simulink model "Project1_week3_sim"  (R2023b)
settings: Solver=VariableStepAuto  StartTime=0.0  StopTime=25  RelTol=1e-7
values from neighbouring files (symbols this model uses):
  A = A_initial(A_index)    [P1_week3_code.m]
  b = b_initial(b_index)    [P1_week3_code.m]
  frequency = 0    [P1_week3_code.m]
  J = J_initial(J_index)    [P1_week3_code.m]
  w_0 = w_0_initial(w_0_index)    [P1_week3_code.m]
settings Model: Creator=rahma  LastModifiedBy=xavie

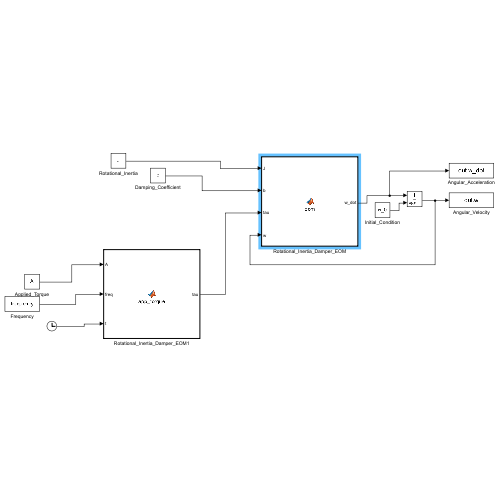
[thumbnail: Simulink's stored preview of the top-level diagram]
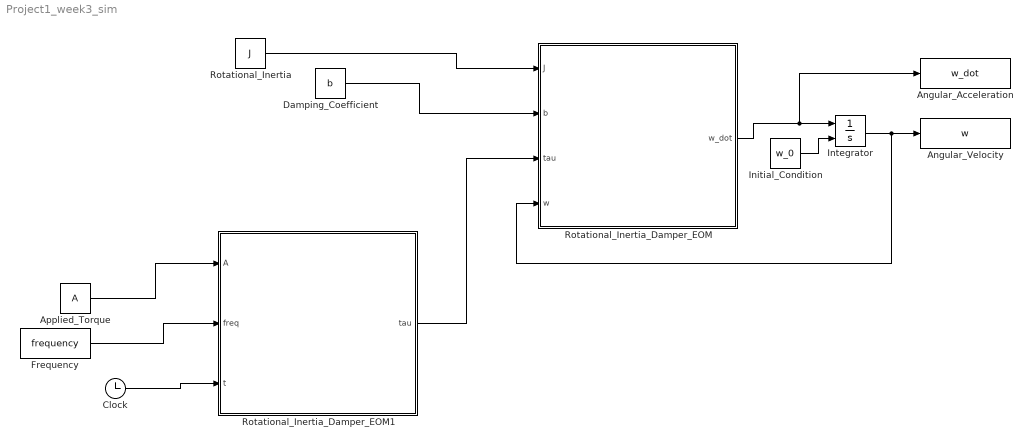
== system Project1_week3_sim ==
  Angular_Acceleration : ToWorkspace  VariableName=w_dot  SaveFormat=Timeseries  SampleTime=-1
  Angular_Velocity : ToWorkspace  VariableName=w  SaveFormat=Timeseries  SampleTime=-1
  Applied_Torque : Constant  Value=A
  Clock : Clock
  Damping_Coefficient : Constant  Value=b
  Frequency : Constant  Value=frequency
  Initial_Condition : Constant  Value=w_0
  Integrator : Integrator  InitialConditionSource=external  ContinuousStateAttributes="\"AngularVelocity\""
  Rotational_Inertia : Constant  Value=J
  Rotational_Inertia_Damper_EOM : MATLAB Function  TreatAsAtomicUnit=on
  Rotational_Inertia_Damper_EOM1 : MATLAB Function  TreatAsAtomicUnit=on
  wires:
  Initial_Condition/1 -> Integrator/2
  Rotational_Inertia_Damper_EOM/1(w_dot) -> Angular_Acceleration/1, Integrator/1
  Damping_Coefficient/1 -> Rotational_Inertia_Damper_EOM/2(b)
  Rotational_Inertia/1 -> Rotational_Inertia_Damper_EOM/1(J)
  Integrator/1 -> Rotational_Inertia_Damper_EOM/4(w), Angular_Velocity/1
  Applied_Torque/1 -> Rotational_Inertia_Damper_EOM1/1(A)
  Clock/1 -> Rotational_Inertia_Damper_EOM1/3(t)
  Rotational_Inertia_Damper_EOM1/1(tau) -> Rotational_Inertia_Damper_EOM/3(tau)
  Frequency/1 -> Rotational_Inertia_Damper_EOM1/2(freq)

== matlab function Project1_week3_sim/Rotational_Inertia_Damper_EOM1 ==
  data: A input; freq input; tau output; t input
function tau = app_torque(A, freq, t) % recieving values
if freq == 0 % since sine wave only happens if there is a frequency 
    tau = A; 
else 
    tau = A.*sin(freq.*t);
end

== matlab function Project1_week3_sim/Rotational_Inertia_Damper_EOM ==
  data: J input; w_dot output; b input; tau input; w input
function w_dot = eom(J, b, tau, w)
% Recall EOM: J*w_dot = tau_applied - tau_damped
tau_damped = b*w;
w_dot = (1/J)*(tau - tau_damped);
%tau_damped = b*w;
% tau = A.*sin(freq.*t);
%w_dot = (1/J).*(tau - tau_damped);
%end
